simulink model "CruiseControlSimulation"  (R2026a)
settings: Solver=VariableStepAuto  StopTime=120
settings Model: Creator=Elsa Lokaj  LastModifiedBy=Elsa Lokaj

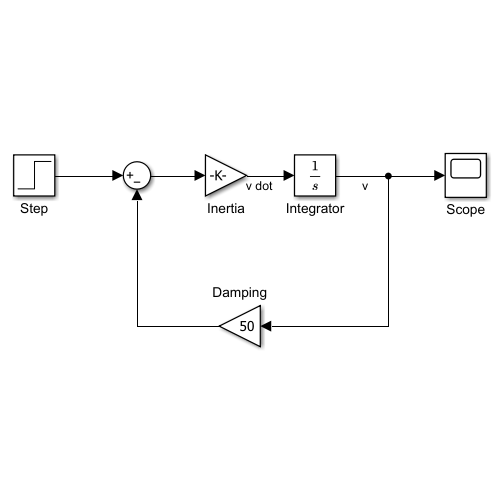
[thumbnail: Simulink's stored preview of the top-level diagram]
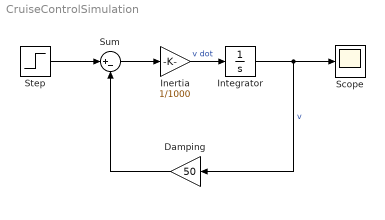
== system CruiseControlSimulation ==
  Damping : Gain  Gain=50
  Inertia : Gain  Gain=1/1000
  Integrator : Integrator
  Scope : Scope
      settings: ActiveDisplayYMinimum=-1.2467426991900008  ActiveDisplayYMaximum=11.220684292710009
  Step : Step  FinalValue=500  SampleTime=0
  Sum : Sum  Inputs=|+-
  wires:
  Inertia/1 -> Integrator/1  "v dot"
  Integrator/1 -> Scope/1, Damping/1  "v"
  Sum/1 -> Inertia/1
  Damping/1 -> Sum/2
  Step/1 -> Sum/1
